simulink library "ctrl_lib"  (R2018a)
settings: Solver=VariableStepAuto  StartTime=0.0  StopTime=10.0  RelTol=1e-3
undefined symbols (not defined in the file): DiscIntNeverNeededParam
libraries: $bdroot x5, peTransforms x1
settings Model: Creator=uids8840  LastModifiedBy=elrobotista
settings CodeAppCC: StateflowObjectComments=on

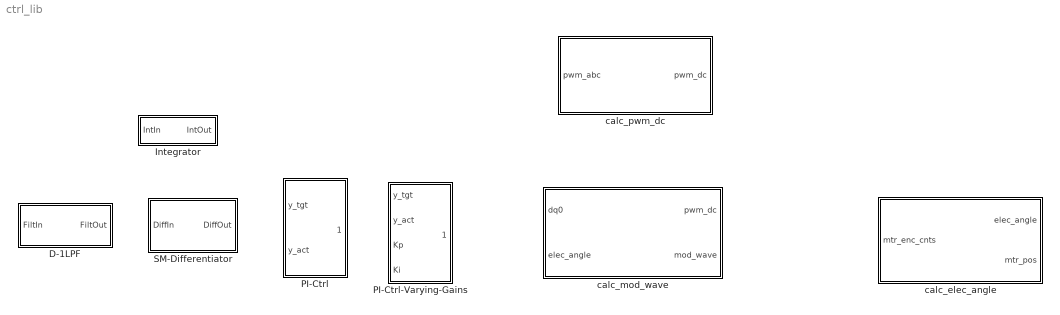
== system ctrl_lib ==
  D-1LPF : Subsystem  mask{k_filt=0.9615}
      mask prompts: k_filt "Filter Constant [tau / (tau + Ts)]:"
      mask DialogControl DescTextVar Prompt: Digital first order low pass filter.
  Integrator : Subsystem  SystemSampleTime=ts  mask{ts=1, max_lim=inf, min_lim=-inf}
      mask prompts: ts "Execution Rate [s]:"; max_lim "Max:"; min_lim "Min:"
      mask DialogControl DescTextVar Prompt: ODE-1 Integrator.
  PI-Ctrl : Subsystem  SystemSampleTime=ts  mask{ts=1, PI_Kp=0, PI_Ki=0, max_lim=inf, min_lim=-inf}
      mask prompts: ts "Execution Rate [s]:"; PI_Kp "Proportional Gain:"; PI_Ki "Integral Gain:"; max_lim "Upper limit"; min_lim "Lower limit"
      mask DialogControl DescTextVar Prompt: Discrete PI Controller.
  PI-Ctrl-Varying-Gains : Subsystem  TreatAsAtomicUnit=on  RTWFcnName=PI_Ctrl  mask{ts=1, max_lim=inf, min_lim=-inf}
      mask prompts: ts "Execution Rate [s]:"; max_lim "Upper limit"; min_lim "Lower limit"
      settings: RTWFcnNameOpts=User specified
      mask DialogControl DescTextVar Prompt: Discrete PI Controller.
  SM-Differentiator : Subsystem  mask{sm_ki=1000, sm_kp=100, ts=1}
      mask prompts: sm_ki "Integral Gain:"; sm_kp "Proportional Gain:"; ts "Execution Rate [s]:"
      mask DialogControl DescTextVar Prompt: Second order sliding mode differentiator.
  calc_elec_angle : Subsystem  TreatAsAtomicUnit=on  mask{n_poles=12, enc_cnts_int=20000}
      mask prompts: n_poles "Number of poles:"; enc_cnts_int "Encoder PPR"
      settings: RTWFcnNameOpts=Use subsystem name
  calc_mod_wave : Subsystem  TreatAsAtomicUnit=on
      settings: RTWFcnNameOpts=Use subsystem name
  calc_pwm_dc : Subsystem  TreatAsAtomicUnit=on
      settings: RTWFcnNameOpts=Use subsystem name

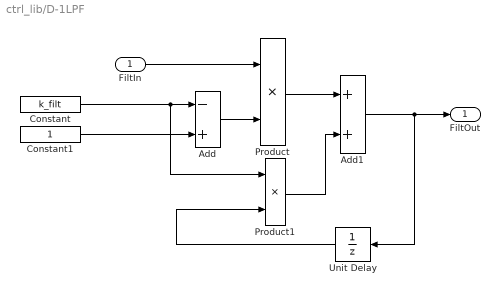
== system ctrl_lib/D-1LPF ==
  FiltIn : Inport
  Add : Sum  Inputs=-+
  Add1 : Sum
  Constant : Constant  Value=k_filt  OutDataTypeStr=Inherit: Inherit via back propagation
  Constant1 : Constant  OutDataTypeStr=Inherit: Inherit via back propagation
  Product : Product  OutDataTypeStr=Inherit: Same as first input
  Product1 : Product  OutDataTypeStr=Inherit: Same as first input
  Unit Delay : UnitDelay  SampleTime=-1
  FiltOut : Outport
  wires:
  Add1/1 -> FiltOut/1, Unit Delay/1
  FiltIn/1 -> Product/1
  Add/1 -> Product/2
  Product/1 -> Add1/1
  Unit Delay/1 -> Product1/2
  Constant/1 -> Product1/1, Add/1
  Constant1/1 -> Add/2
  Product1/1 -> Add1/2

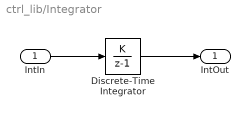
== system ctrl_lib/Integrator ==
  IntIn : Inport
  Discrete-Time Integrator : DiscreteIntegrator  IntegratorMethod=Accumulation: Forward Euler  gainval=ts  SampleTime=-1  LimitOutput=on  UpperSaturationLimit=max_lim  LowerSaturationLimit=min_lim  ICPrevOutput=DiscIntNeverNeededParam  ICPrevScaledInput=DiscIntNeverNeededParam
  IntOut : Outport
  wires:
  IntIn/1 -> Discrete-Time Integrator/1
  Discrete-Time Integrator/1 -> IntOut/1

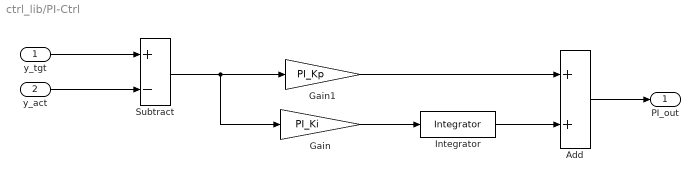
== system ctrl_lib/PI-Ctrl ==
  y_tgt : Inport
  y_act : Inport  Port=2
  Add : Sum  OutDataTypeStr=Inherit: Inherit via back propagation
  Gain : Gain  Gain=PI_Ki  ParamDataTypeStr=Inherit: Inherit from 'Gain'  OutDataTypeStr=Inherit: Inherit via back propagation
  Gain1 : Gain  Gain=PI_Kp  ParamDataTypeStr=Inherit: Inherit from 'Gain'  OutDataTypeStr=Inherit: Inherit via back propagation
  Integrator : $bdroot/Integrator  ts=ts  max_lim=max_lim  min_lim=min_lim
  Subtract : Sum  Inputs=+-
  PI_out : Outport
  wires:
  y_tgt/1 -> Subtract/1
  Gain1/1 -> Add/1
  y_act/1 -> Subtract/2
  Subtract/1 -> Gain/1, Gain1/1
  Gain/1 -> Integrator/1
  Integrator/1 -> Add/2
  Add/1 -> PI_out/1

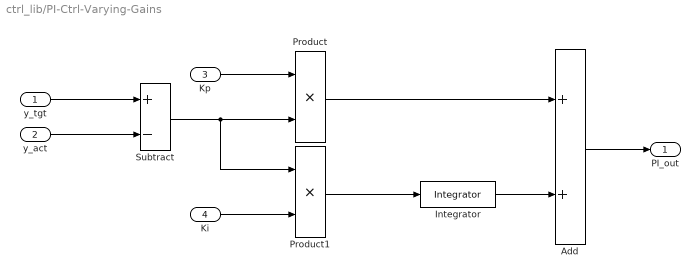
== system ctrl_lib/PI-Ctrl-Varying-Gains ==
  y_tgt : Inport
  y_act : Inport  Port=2
  Kp : Inport  Port=3
  Ki : Inport  Port=4
  Add : Sum  OutDataTypeStr=Inherit: Inherit via back propagation
  Integrator : $bdroot/Integrator  ts=ts  max_lim=max_lim  min_lim=min_lim
  Product : Product
  Product1 : Product
  Subtract : Sum  Inputs=+-
  PI_out : Outport
  wires:
  Add/1 -> PI_out/1
  Integrator/1 -> Add/2
  Product1/1 -> Integrator/1
  Subtract/1 -> Product1/1, Product/2
  y_act/1 -> Subtract/2
  Product/1 -> Add/1
  y_tgt/1 -> Subtract/1
  Kp/1 -> Product/1
  Ki/1 -> Product1/2

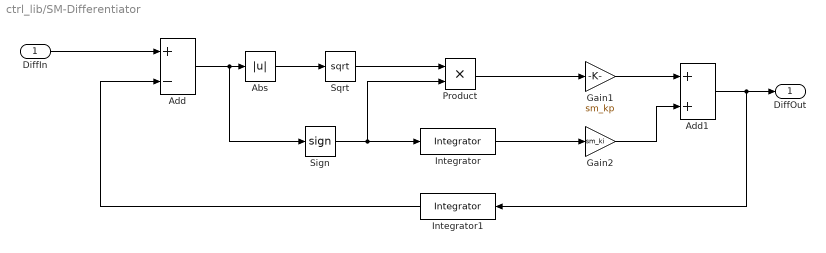
== system ctrl_lib/SM-Differentiator ==
  DiffIn : Inport
  Abs : Abs
  Add : Sum  Inputs=+-
  Add1 : Sum  OutDataTypeStr=Inherit: Inherit via back propagation
  Gain1 : Gain  Gain=sm_kp  ParamDataTypeStr=Inherit: Inherit from 'Gain'  OutDataTypeStr=Inherit: Inherit via back propagation
  Gain2 : Gain  Gain=sm_ki  ParamDataTypeStr=Inherit: Inherit from 'Gain'  OutDataTypeStr=Inherit: Inherit via back propagation
  Integrator : $bdroot/Integrator  ts=ts
  Integrator1 : $bdroot/Integrator  ts=ts
  Product : Product  OutDataTypeStr=Inherit: Same as first input
  Sign : Signum
  Sqrt : Sqrt  SaturateOnIntegerOverflow=on
  DiffOut : Outport
  wires:
  Gain2/1 -> Add1/2
  Integrator1/1 -> Add/2
  Sign/1 -> Integrator/1, Product/2
  Sqrt/1 -> Product/1
  Add1/1 -> Integrator1/1, DiffOut/1
  DiffIn/1 -> Add/1
  Abs/1 -> Sqrt/1
  Gain1/1 -> Add1/1
  Integrator/1 -> Gain2/1
  Product/1 -> Gain1/1
  Add/1 -> Sign/1, Abs/1

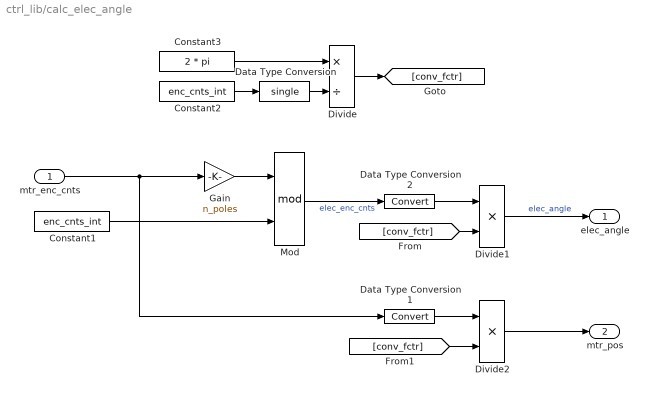
== system ctrl_lib/calc_elec_angle ==
  mtr_enc_cnts : Inport
  Constant1 : Constant  Value=enc_cnts_int
  Constant2 : Constant  Value=enc_cnts_int
  Constant3 : Constant  Value=2 * pi  OutDataTypeStr=single
  Data Type Conversion : DataTypeConversion  OutDataTypeStr=single  RndMeth=Simplest
  Data Type Conversion1 : DataTypeConversion
  Data Type Conversion2 : DataTypeConversion
  Divide : Product  Inputs=*/
  Divide1 : Product  Inputs=**
  Divide2 : Product  Inputs=**
  Gain : Gain  Gain=n_poles  ParamDataTypeStr=int32  OutDataTypeStr=int32
      settings: AttributesFormatString=%<Gain>
  Mod : Math  Operator=mod  SaturateOnIntegerOverflow=on
  elec_angle : Outport
  mtr_pos : Outport  Port=2
  wires:
  Divide1/1 -> elec_angle/1  "elec_angle"
  Divide2/1 -> mtr_pos/1
  Mod/1 -> Data Type Conversion2/1  "elec_enc_cnts"
  Gain/1 -> Mod/1
  mtr_enc_cnts/1 -> Gain/1, Data Type Conversion1/1
  Data Type Conversion1/1 -> Divide2/1
  Data Type Conversion2/1 -> Divide1/1
  Constant1/1 -> Mod/2
  Constant2/1 -> Data Type Conversion/1
  Constant3/1 -> Divide/1
  Data Type Conversion/1 -> Divide/2
  Divide/1 -> [conv_fctr]
  [conv_fctr] -> Divide1/2
  [conv_fctr] -> Divide2/2

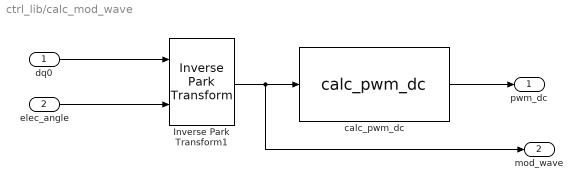
== system ctrl_lib/calc_mod_wave ==
  dq0 : Inport
  elec_angle : Inport  Port=2
  Inverse Park Transform1 : peTransforms/Inverse Park Transform  AxisAlignment=D-axis  PowerInvariant=off
  calc_pwm_dc : $bdroot/calc_pwm_dc
  pwm_dc : Outport
  mod_wave : Outport  Port=2
  wires:
  Inverse Park Transform1/1 -> calc_pwm_dc/1, mod_wave/1
  elec_angle/1 -> Inverse Park Transform1/2
  dq0/1 -> Inverse Park Transform1/1
  calc_pwm_dc/1 -> pwm_dc/1

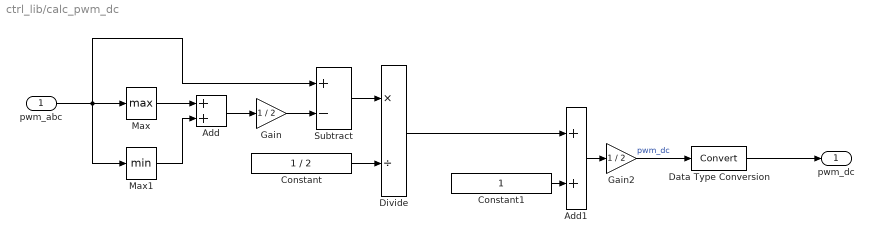
== system ctrl_lib/calc_pwm_dc ==
  pwm_abc : Inport
  Add : Sum
  Add1 : Sum
  Constant : Constant  Value=1 / 2  OutDataTypeStr=Inherit: Inherit via back propagation
  Constant1 : Constant  OutDataTypeStr=Inherit: Inherit via back propagation
  Data Type Conversion : DataTypeConversion
  Divide : Product  Inputs=*/
  Gain : Gain  Gain=1 / 2
      settings: AttributesFormatString=%<Gain>
  Gain2 : Gain  Gain=1 / 2
      settings: AttributesFormatString=%<Gain>
  Max : MinMax  Function=max
  Max1 : MinMax
  Subtract : Sum  Inputs=+-
  pwm_dc : Outport  VectorParamsAs1DForOutWhenUnconnected=on
  wires:
  Data Type Conversion/1 -> pwm_dc/1
  Gain2/1 -> Data Type Conversion/1  "pwm_dc"
  Add1/1 -> Gain2/1
  Constant1/1 -> Add1/2
  Divide/1 -> Add1/1
  Constant/1 -> Divide/2
  Subtract/1 -> Divide/1
  Gain/1 -> Subtract/2
  Add/1 -> Gain/1
  Max1/1 -> Add/2
  Max/1 -> Add/1
  pwm_abc/1 -> Max/1, Max1/1, Subtract/1
